simulink model "Sistema_LTI"  (R2023a)
settings: Solver=VariableStepAuto  StartTime=0.0  StopTime=10.0  RelTol=1e-3
undefined symbols (not defined in the file): b_eq, C_ts, J_eq, k_l, L_q, lambda_m, Pp, r, R_s_ref, R_ts
settings Model: Creator=juanf  LastModifiedBy=juanf

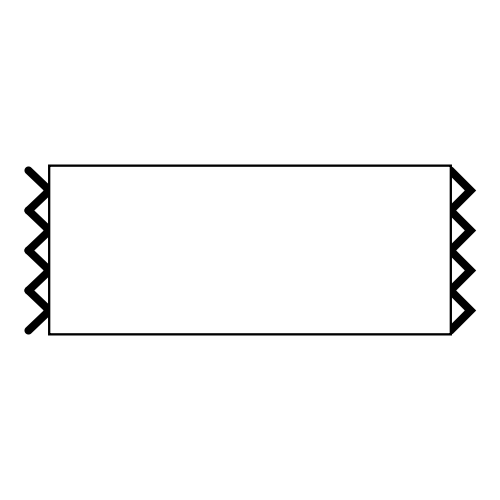
[thumbnail: Simulink's stored preview of the top-level diagram]
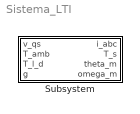
== system Sistema_LTI ==
  Subsystem : Subsystem

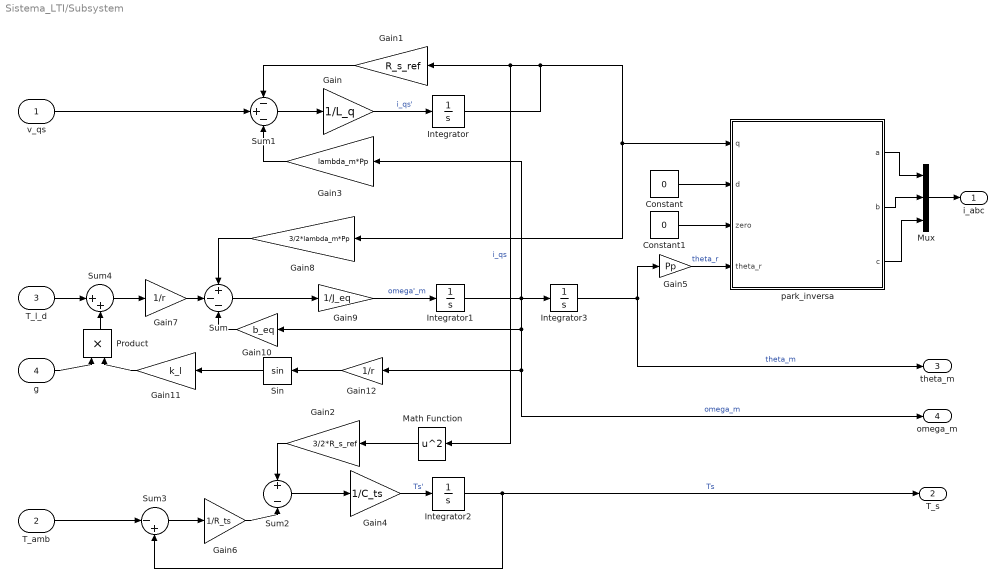
== system Sistema_LTI/Subsystem ==
  v_qs : Inport
  T_amb : Inport  Port=2
  T_l_d : Inport  Port=3
  g : Inport  Port=4
  Constant : Constant  Value=0
  Constant1 : Constant  Value=0
  Gain : Gain  Gain=1/L_q
  Gain1 : Gain  Gain=R_s_ref
  Gain10 : Gain  Gain=b_eq
  Gain11 : Gain  Gain=k_l
  Gain12 : Gain  Gain=1/r
  Gain2 : Gain  Gain=3/2*R_s_ref
  Gain3 : Gain  Gain=lambda_m*Pp
  Gain4 : Gain  Gain=1/C_ts
  Gain5 : Gain  Gain=Pp
  Gain6 : Gain  Gain=1/R_ts
  Gain7 : Gain  Gain=1/r
  Gain8 : Gain  Gain=3/2*lambda_m*Pp
  Gain9 : Gain  Gain=1/J_eq
  Integrator{,1..3} (4 alike) : Integrator
  Math Function : Math  Operator=square  SignedPower=on
  Mux : Mux  Inputs=3
  Product : Product
  Sin : Trigonometry
  Sum : Sum  Inputs=+--
  Sum1 : Sum  Inputs=-+-
  Sum2 : Sum  Inputs=+|-
  Sum3 : Sum  Inputs=|-+
  Sum4 : Sum  Inputs=|++
  park_inversa : MATLAB Function  TreatAsAtomicUnit=on
  i_abc : Outport
  T_s : Outport  Port=2
  theta_m : Outport  Port=3
  omega_m : Outport  Port=4
  wires:
  Constant/1 -> park_inversa/2(d)
  Constant1/1 -> park_inversa/3(zero)
  park_inversa/1(a) -> Mux/1
  park_inversa/2(b) -> Mux/2
  park_inversa/3(c) -> Mux/3
  Gain/1 -> Integrator/1  "i_qs'"
  Integrator/1 -> Gain1/1, Math Function/1, park_inversa/1(q), Gain8/1  "i_qs"
  v_qs/1 -> Sum1/2
  Gain1/1 -> Sum1/1
  Sum1/1 -> Gain/1
  Gain3/1 -> Sum1/3
  Gain6/1 -> Sum2/2
  Gain2/1 -> Sum2/1
  Math Function/1 -> Gain2/1
  Sum2/1 -> Gain4/1
  Gain4/1 -> Integrator2/1  "Ts'"
  Integrator2/1 -> Sum3/2, T_s/1  "Ts"
  Sum3/1 -> Gain6/1
  Mux/1 -> i_abc/1
  Gain7/1 -> Sum/2
  Gain8/1 -> Sum/1
  Sum/1 -> Gain9/1
  Gain9/1 -> Integrator1/1  "omega'_m"
  Integrator1/1 -> Gain12/1, omega_m/1, Gain10/1, Integrator3/1, Gain3/1  "omega_m"
  Gain10/1 -> Sum/3
  Integrator3/1 -> Gain5/1, theta_m/1  "theta_m"
  Gain5/1 -> park_inversa/4(theta_r)  "theta_r"
  T_amb/1 -> Sum3/1
  Sum4/1 -> Gain7/1
  T_l_d/1 -> Sum4/1
  Gain11/1 -> Product/2
  Sin/1 -> Gain11/1
  Gain12/1 -> Sin/1
  Product/1 -> Sum4/2
  g/1 -> Product/1

== matlab function Sistema_LTI/Subsystem/park_inversa ==
  data: q input; a output; d input; zero input; theta_r input; b output; c output
function [a, b, c] = park_inversa(q, d, zero, theta_r)
% qd0 → abc (transformacion inversa)
% Entradas: q, d, zero (coordenadas qd0), theta_r (ángulo eléctrico)
% Salidas: a, b, c (señales de fase)
    
    T_inv = [cos(theta_r),               sin(theta_r),              1;
             cos(theta_r - 2*pi/3),      sin(theta_r - 2*pi/3),     1;
             cos(theta_r + 2*pi/3),      sin(theta_r + 2*pi/3),     1];
    
    abc = T_inv * [q; d; zero];

    a = abc(1);
    b = abc(2);
    c = abc(3);
end
